simulink model "Q2_Model"  (R2021a)
settings: Solver=ode8  StartTime=0.0  StopTime=60  FixedStep=1e-4  RelTol=1e-3
InitFcn:
  | MagicFormula
  | LookUpTable
  | Q2_constants
values from neighbouring files (symbols this model uses):
  engine_torque = [-40 -44 -49 -53 -57 -61 -65 -70 -74 -78 -82 ... (first row only)    [LookUpTable.m]
  Je = 0.7    [Q2_constants.m]
  Jw = 0.7    [Q2_constants.m]
  MagicTire_Fx = Fx    [MagicFormula.m]
  MagicTire_Fy = Fy    [MagicFormula.m]
  MagicTire_Fz = 2000:2000:8000    [MagicFormula.m]
  Reff = 0.315    [Q2_constants.m]
  throt_angle = [0, 20, 30, 40, 50, 60, 70, 80, 90, 100]    [LookUpTable.m]
  whel_rot_angle = [83.70, 125.6, 167.5, 209.4, 251.3, 293.2, 335.1, 377.0, 418.9, 460.7, 502.6]    [LookUpTable.m]
undefined symbols (not defined in the file or in its folder): sigbuilder_block
libraries: pid_lib x1
settings Model: Creator=Fatih  LastModifiedBy=Fatih
settings DataIOCC: ReturnWorkspaceOutputs=off

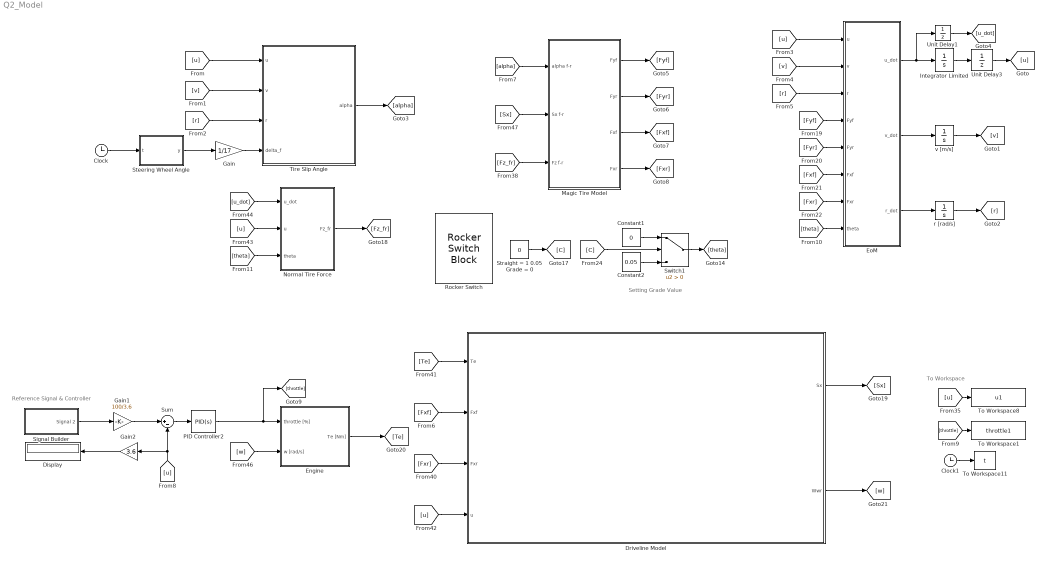
== system Q2_Model ==
  note: Reference Signal & Controller
  note: To Workspace
  note: Setting Grade Value
  Clock : Clock
  Clock1 : Clock
  Constant1 : Constant  Value=0
  Constant2 : Constant  Value=0.05
  Display : Display
  Driveline Model : Subsystem
  Engine : Subsystem
  EoM : MATLAB Function  TreatAsAtomicUnit=on
  Gain : Gain  Gain=1/17
  Gain1 : Gain  Gain=100/3.6
  Gain2 : Gain  Gain=3.6
  Integrator Limited : Integrator  InitialCondition=60/3.6  LimitOutput=on  UpperSaturationLimit=500  LowerSaturationLimit=1
  Magic Tire Model : Subsystem
  Normal Tire Force : MATLAB Function  TreatAsAtomicUnit=on
  PID Controller2 : pid_lib/PID Controller  Controller=PID  Form=Parallel  TimeDomain=Continuous-time  UseExternalTs=off  SampleTime=-1  IntegratorMethod=Forward Euler  FilterMethod=Forward Euler  ControllerParametersSource=internal  P=11  I=0.12  D=4  UseFilter=on  N=100  TunerSelectOption=Frequency Response Based  InitialConditionSource=internal  InitialConditionForIntegrator=0  InitialConditionForFilter=0  DifferentiatorICPrevScaledInput=0  ExternalReset=none  TrackingMode=off  Kt=1  LimitOutput=on  SatLimitsSource=internal  UpperSaturationLimit=90  LowerSaturationLimit=0  LinearizeAsGain=on  AntiWindupMode=none  Kb=1  POutMin=[]  POutMax=[]  IOutMin=[]  IOutMax=[]  DOutMin=[]  DOutMax=[]  NOutMin=[]  NOutMax=[]  SumOutMin=[]  SumOutMax=[]  SaturationOutMin=[]  SaturationOutMax=[]  PParamMin=[]  PParamMax=[]  IParamMin=[]  IParamMax=[]  DParamMin=[]  DParamMax=[]  NParamMin=[]  NParamMax=[]  KbParamMin=[]  KbParamMax=[]  KtParamMin=[]  KtParamMax=[]  KbOutMin=[]  KbOutMax=[]  KtOutMin=[]  KtOutMax=[]  IntegratorOutMin=[]  IntegratorOutMax=[]  FilterOutMin=[]  FilterOutMax=[]  SumI1OutMin=[]  SumI1OutMax=[]  SumI2OutMin=[]  SumI2OutMax=[]  SumI3OutMin=[]  SumI3OutMax=[]  SumI4OutMin=[]  SumI4OutMax=[]  SumDOutMin=[]  SumDOutMax=[]  DifferentiatorOutMin=[]  DifferentiatorOutMax=[]  FilterDiffOutCoefMin=[]  FilterDiffOutCoefMax=[]  ReciprocalOutMin=[]  ReciprocalOutMax=[]  SumDenOutMin=[]  SumDenOutMax=[]  SumNumOutMin=[]  SumNumOutMax=[]  DivideOutMin=[]  DivideOutMax=[]  UdiffTsProdOutMin=[]  UdiffTsProdOutMax=[]  NTsProdOutMin=[]  NTsProdOutMax=[]  UintegralTsProdOutMin=[]  UintegralTsProdOutMax=[]  UngainTsProdOutMin=[]  UngainTsProdOutMax=[]  IntegratorContinuousStateAttributes=''  IntegratorStateMustResolveToSignalObject=off  IntegratorRTWStateStorageClass=Auto  FilterContinuousStateAttributes=''  FilterStateMustResolveToSignalObject=off  FilterRTWStateStorageClass=Auto  ParallelPVariant=InternalParameters  IdealPVariant=Disabled  IVariant=InternalParameters  DVariant=InternalParameters  IntegratorVariant=Continuous  SatVariant=Enabled  AWVariant=Passthrough  PCopyVariant=Disabled  TRVariant=Disabled  FdbkBlocksVariant=Forward  IdealPFdbkVariant=Disabled  SatFdbkVariant=Disabled  DerivativeFilterVariant=ContFilter  NVariant=InternalParameters  NCopyVariant=Disabled  FilterICVariant=InternalICsFilter  IntegratorICVariant=InternalICs  ExternalResetVariant=Disabled  TRSumVariant=Passthrough  SumFdbkVariant=Disabled  SumVariant=Sum_PID  TsampFilterVariant=InternalTs  TsampNgainVariant=Passthrough  TsampIntegralVariant=Passthrough  ExternalSaturationOutDataTypeStr=Inherit: Same as second input
  Rocker Switch : RockerSwitchBlock
      settings: Values={{'Off', 'On'}, [0 1]}
  Signal Builder : Subsystem  Tag=STV Subsys  LoadFcn=sigbuilder_block('load');  StartFcn=sigbuilder_block('start');  StopFcn=sigbuilder_block('stop');  ClipboardFcn=sigbuilder_block('clipboard');  mask(Sigbuilder block){tuvar=[0:10]}
      mask help: Simulink:masks:SigbuilderBlock_MD
      mask init:
      | if ~strcmp(get_param(bdroot(gcbh),'SimulationStatus'),'stopped') tuvar = sigbuilder_block('maskInit'); end
      settings: CopyFcn=sigbuilder_block('copy');  DeleteFcn=sigbuilder_block('delete');  ModelCloseFcn=sigbuilder_block('modelClose');  PreSaveFcn=sigbuilder_block('preSave');  PauseFcn=sigbuilder_block('pause');  ContinueFcn=sigbuilder_block('continue');  NameChangeFcn=sigbuilder_block('namechange');  OpenFcn=sigbuilder_block('open',[437.6 199.2 550.4 400 ]);  CloseFcn=sigbuilder_block('close');
      mask Display: plot(0, 0, 100, 100,[2, 2, 32, 32, 2], [68, 8, 8, 68, 68],[32, 2], [38, 38], [32, 19, 2],[53, 60, 44], [32, 17, 17, 2],[16, 16, 31, 31]);txt = getActiveGroup(gcbh);text(2, 100, txt,'verticalAlignment', 'top');
  Steering Wheel Angle : MATLAB Function  TreatAsAtomicUnit=on
  Straight = 1 0.05 Grade = 0 : Constant  Value=0
  Sum : Sum  Inputs=|+-
  Switch1 : Switch  Criteria=u2 > Threshold
  Tire Slip Angle : MATLAB Function  TreatAsAtomicUnit=on
  To Workspace1 : ToWorkspace  VariableName=throttle1  SaveFormat=Timeseries  SampleTime=-1
      settings: Save2DSignal=2-D array (concatenate along first dimension)
  To Workspace11 : ToWorkspace  VariableName=t  SampleTime=-1
      settings: Save2DSignal=2-D array (concatenate along first dimension)
  To Workspace8 : ToWorkspace  VariableName=u1  SaveFormat=Timeseries  SampleTime=-1
      settings: Save2DSignal=2-D array (concatenate along first dimension)
  Unit Delay1 : UnitDelay  InitialCondition=1  SampleTime=-1  HasFrameUpgradeWarning=on
  Unit Delay3 : UnitDelay  InitialCondition=1  SampleTime=-1  HasFrameUpgradeWarning=on
  r [rad/s] : Integrator  InitialCondition=0.001
  v [m/s] : Integrator
  wires:
  Gain/1 -> Tire Slip Angle/4(delta_f)
  EoM/2(v_dot) -> v [m/s]/1
  EoM/3(r_dot) -> r [rad/s]/1
  v [m/s]/1 -> [v]
  r [rad/s]/1 -> [r]
  [u] -> Tire Slip Angle/1(u)
  [v] -> Tire Slip Angle/2(v)
  [r] -> Tire Slip Angle/3(r)
  [u] -> EoM/1(u)
  [r] -> EoM/3(r)
  Integrator Limited/1 -> Unit Delay3/1
  Clock/1 -> Steering Wheel Angle/1(t)
  Steering Wheel Angle/1(y) -> Gain/1
  Engine/1(Te [Nm]) -> [Te]
  Tire Slip Angle/1(alpha) -> [alpha]
  [alpha] -> Magic Tire Model/1(alpha f-r)
  [Sx] -> Magic Tire Model/2(Sx f-r)
  Magic Tire Model/3(Fxf) -> [Fxf]
  Magic Tire Model/2(Fyr) -> [Fyr]
  Magic Tire Model/1(Fyf) -> [Fyf]
  [Fyf] -> EoM/4(Fyf)
  [Fyr] -> EoM/5(Fyr)
  [Fxf] -> EoM/6(Fxf)
  [Fxr] -> EoM/7(Fxr)
  [u] -> To Workspace8/1
  Clock1/1 -> To Workspace11/1
  [Fz_fr] -> Magic Tire Model/3(Fz f-r)
  Magic Tire Model/4(Fxr) -> [Fxr]
  [w] -> Engine/2(w [rad/s])
  Unit Delay3/1 -> [u]
  [u] -> Sum/2, Gain2/1
  Signal Builder/1(Signal 2) -> Gain1/1
  Gain1/1 -> Sum/1
  Gain2/1 -> Display/1
  [Te] -> Driveline Model/1(Te)
  [Fxf] -> Driveline Model/2(Fxf)
  [Fxr] -> Driveline Model/3(Fxr)
  [u] -> Driveline Model/4(u)
  Driveline Model/1(Sx) -> [Sx]
  Driveline Model/2(Wwr) -> [w]
  [u] -> Normal Tire Force/2(u)
  [u_dot] -> Normal Tire Force/1(u_dot)
  Normal Tire Force/1(Fz_fr) -> [Fz_fr]
  PID Controller2/1 -> [throttle], Engine/1(throttle [%])
  Sum/1 -> PID Controller2/1
  EoM/1(u_dot) -> Unit Delay1/1, Integrator Limited/1
  Unit Delay1/1 -> [u_dot]
  [throttle] -> To Workspace1/1
  [v] -> EoM/2(v)
  Switch1/1 -> [theta]
  Constant2/1 -> Switch1/3
  [C] -> Switch1/2
  Straight = 1 0.05 Grade = 0/1 -> [C]
  Constant1/1 -> Switch1/1
  [theta] -> EoM/8(theta)
  [theta] -> Normal Tire Force/3(theta)

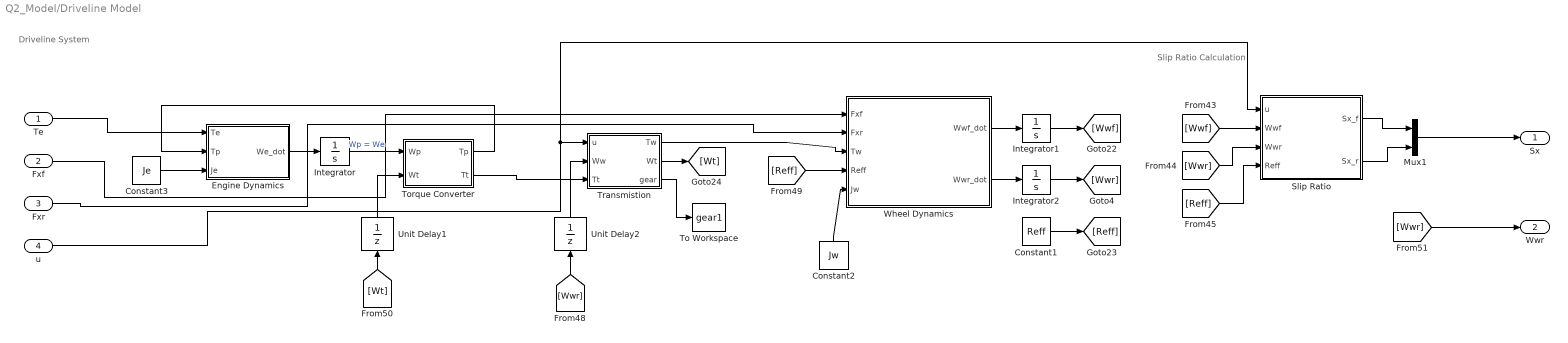
== system Q2_Model/Driveline Model ==
  note: Slip Ratio Calculation
  note: Driveline System
  Te : Inport
  Fxf : Inport  Port=2
  Fxr : Inport  Port=3
  u : Inport  Port=4
  Constant1 : Constant  Value=Reff
  Constant2 : Constant  Value=Jw
  Constant3 : Constant  Value=Je
  Engine Dynamics : MATLAB Function  TreatAsAtomicUnit=on
  Integrator : Integrator
  Integrator1 : Integrator  InitialCondition=100
  Integrator2 : Integrator  InitialCondition=100
  Mux1 : Mux  Inputs=2
  Slip Ratio : MATLAB Function  TreatAsAtomicUnit=on
  To Workspace : ToWorkspace  VariableName=gear1  SaveFormat=Timeseries  SampleTime=-1
  Torque Converter : MATLAB Function  TreatAsAtomicUnit=on
  Transmistion : MATLAB Function  TreatAsAtomicUnit=on
  Unit Delay1 : UnitDelay  InitialCondition=1  SampleTime=-1  HasFrameUpgradeWarning=on
  Unit Delay2 : UnitDelay  InitialCondition=1  SampleTime=-1  HasFrameUpgradeWarning=on
  Wheel Dynamics : MATLAB Function  TreatAsAtomicUnit=on
  Sx : Outport
  Wwr : Outport  Port=2
  wires:
  Engine Dynamics/1(We_dot) -> Integrator/1
  [Reff] -> Wheel Dynamics/4(Reff)
  [Wt] -> Unit Delay1/1
  u/1 -> Transmistion/1(u), Slip Ratio/1(u)
  [Wwr] -> Unit Delay2/1
  Integrator1/1 -> [Wwf]
  Unit Delay2/1 -> Transmistion/2(Ww)
  Transmistion/2(Wt) -> [Wt]
  Integrator2/1 -> [Wwr]
  Slip Ratio/1(Sx_f) -> Mux1/1
  Integrator/1 -> Torque Converter/1(Wp)  "Wp = We"
  [Wwf] -> Slip Ratio/2(Wwf)
  Slip Ratio/2(Sx_r) -> Mux1/2
  Constant1/1 -> [Reff]
  Unit Delay1/1 -> Torque Converter/2(Wt)
  Constant2/1 -> Wheel Dynamics/5(Jw)
  Fxr/1 -> Wheel Dynamics/2(Fxr)
  Wheel Dynamics/2(Wwr_dot) -> Integrator2/1
  [Wwr] -> Slip Ratio/3(Wwr)
  Torque Converter/1(Tp) -> Engine Dynamics/2(Tp)
  Transmistion/1(Tw) -> Wheel Dynamics/3(Tw)
  Constant3/1 -> Engine Dynamics/3(Je)
  [Reff] -> Slip Ratio/4(Reff)
  Wheel Dynamics/1(Wwf_dot) -> Integrator1/1
  Mux1/1 -> Sx/1
  [Wwr] -> Wwr/1
  Fxf/1 -> Wheel Dynamics/1(Fxf)
  Te/1 -> Engine Dynamics/1(Te)
  Transmistion/3(gear) -> To Workspace/1
  Torque Converter/2(Tt) -> Transmistion/3(Tt)

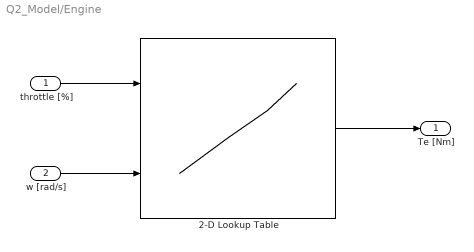
== system Q2_Model/Engine ==
  throttle [%] : Inport
  w [rad/s] : Inport  Port=2
  2-D Lookup Table : Lookup_n-D  BreakpointsForDimension1=throt_angle  BreakpointsForDimension2=whel_rot_angle  Table=engine_torque  InternalRulePriority=Speed  RndMeth=Simplest  InputSameDT=on
      settings: InputPortMap=u0,u1
  Te [Nm] : Outport
  wires:
  2-D Lookup Table/1 -> Te [Nm]/1
  throttle [%]/1 -> 2-D Lookup Table/1
  w [rad/s]/1 -> 2-D Lookup Table/2

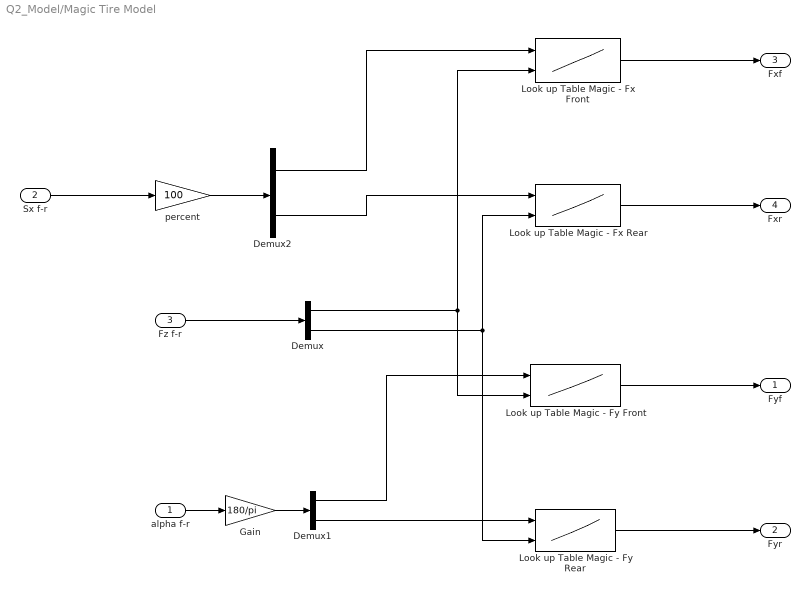
== system Q2_Model/Magic Tire Model ==
  alpha f-r : Inport
  Sx f-r : Inport  Port=2
  Fz f-r : Inport  Port=3
  Demux : Demux  Outputs=2
  Demux1 : Demux  Outputs=2
  Demux2 : Demux  Outputs=2
  Gain : Gain  Gain=180/pi
  Look up Table Magic - Fx Front : Lookup_n-D  BreakpointsForDimension1=MagicTire_slip_ratio'  BreakpointsForDimension2=MagicTire_Fz  Table=MagicTire_Fx  InternalRulePriority=Speed  RndMeth=Simplest  InputSameDT=on
      settings: InputPortMap=u0,u1
  Look up Table Magic - Fx Rear : Lookup_n-D  BreakpointsForDimension1=MagicTire_slip_ratio'  BreakpointsForDimension2=MagicTire_Fz  Table=MagicTire_Fx  InternalRulePriority=Speed  RndMeth=Simplest  InputSameDT=on
      settings: InputPortMap=u0,u1
  Look up Table Magic - Fy Front : Lookup_n-D  BreakpointsForDimension1=MagicTire_alpha'  BreakpointsForDimension2=MagicTire_Fz  Table=MagicTire_Fy  InternalRulePriority=Speed  RndMeth=Simplest  InputSameDT=on
      settings: InputPortMap=u0,u1
  Look up Table Magic - Fy Rear : Lookup_n-D  BreakpointsForDimension1=MagicTire_alpha'  BreakpointsForDimension2=MagicTire_Fz  Table=MagicTire_Fy  InternalRulePriority=Speed  RndMeth=Simplest  InputSameDT=on
      settings: InputPortMap=u0,u1
  percent : Gain  Gain=100
  Fyf : Outport
  Fyr : Outport  Port=2
  Fxf : Outport  Port=3
  Fxr : Outport  Port=4
  wires:
  Gain/1 -> Demux1/1
  Demux/1 -> Look up Table Magic - Fy Front/2, Look up Table Magic - Fx Front/2
  Sx f-r/1 -> percent/1
  alpha f-r/1 -> Gain/1
  Demux1/2 -> Look up Table Magic - Fy Rear/1
  Demux1/1 -> Look up Table Magic - Fy Front/1
  Demux/2 -> Look up Table Magic - Fy Rear/2, Look up Table Magic - Fx Rear/2
  Fz f-r/1 -> Demux/1
  Look up Table Magic - Fx Front/1 -> Fxf/1
  Look up Table Magic - Fx Rear/1 -> Fxr/1
  Look up Table Magic - Fy Front/1 -> Fyf/1
  Look up Table Magic - Fy Rear/1 -> Fyr/1
  percent/1 -> Demux2/1
  Demux2/2 -> Look up Table Magic - Fx Rear/1
  Demux2/1 -> Look up Table Magic - Fx Front/1

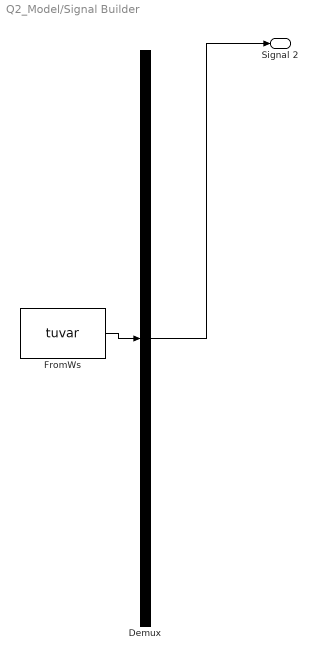
== system Q2_Model/Signal Builder ==
  Demux : Demux  Tag=STV Demux  Outputs=1
      settings: DisplayOption=none
  FromWs : FromWorkspace  Tag=STV FromWs  VariableName=tuvar
      SigBuilderData=|
      | common.afterFinalStr = 'Extrapolate'
      | common.sampleTime = 0
      | dataSet.timeRange = [0 80]
      | dataSet.name = 'Group 1'
      | sbobj.Groups.Name = 'Group 1'
      | sbobj.Groups.Signals.Name = 'Signal 2'
      | sbobj.Groups.Signals.XData = [0 10 10 30 30 80]
      | sbobj.Groups.Signals.YData = [0.6 0.6 1 1 0.4 0.4]
      | sbobj.Groups.TimeRange = [0 80]
  Signal 2 : Outport  Tag=STV Outport
  wires:
  FromWs/1 -> Demux/1
  Demux/1 -> Signal 2/1

== matlab function Q2_Model/Tire Slip Angle ==
  data: u input; alpha output; v input; r input; delta_f input
function alpha  = fcn(u,v,r,delta_f)

%Constants
lf = 1421e-03;  %longitudinal distance from c.g. to FREONT tires
lr = 1029e-03; %longitudinal distance from c.g. to REAR tires


alpha_f = delta_f -((v+lf*r)/u);    %Tire Slip angle front (eq:2.23 and eq:2.29 @ Rajesh Rajamani’s book)

alpha_r =  -((v-lr*r)/u);           %Tire Slip angle rear (eq:2.24 and eq:2.30 @ Rajesh Rajamani’s book)

alpha=[alpha_f,alpha_r];

== matlab function Q2_Model/Normal Tire Force ==
  data: u_dot input; Fz_fr output; u input; theta input
function Fz_fr = fcn(u_dot,u,theta)

% Constants
m = 1480; % kg
g = 9.81; % m/s^2
lf = 1421*10^-3; % m
lr = 1029*10^-3; % m
h_g = 420*10^-3; % m
h_aero = 1.2*h_g; % m (assumption)

rho = 1.225; % kg/m^3
Cd = 0.335;
Area_front = 1.824; % m^2
F_aero = 0.5*rho*Cd*Area_front*u^2;

Fzf = ((-F_aero*h_aero)-(m*u_dot*h_g)-(m*g*h_g*sin(theta))+(m*g*lr*cos(theta)))/(lf+lr);
Fzr = ((F_aero*h_aero)+(m*u_dot*h_g)-(m*g*h_g*sin(theta))+(m*g*lf*cos(theta)))/(lf+lr);

Fz_fr = [Fzf Fzr];

== matlab function Q2_Model/EoM ==
  data: u input; v input; u_dot output; r input; Fyf input; Fyr input; v_dot output; r_dot output; Fxf input; Fxr input; theta input
function [u_dot,v_dot,r_dot] = fcn(u,v,r,Fyf,Fyr,Fxf,Fxr,theta)

%% constants
Jz = 1950;          %[kgm^2]
lf = 1421*10^-3;     %[m] 
lr = 1029*10^-3;    %[m]

%% Aerodynamic Force
rho = 1.225;                        %[kg/m^2]
Cd = 0.335;                          %
Area_front = 1.824;       %[m^2]

% Rolling resistance
m = 1480;                            %[kg]
g = 9.81;                           %[m/s^2]
f0 = 0.013;                         %
Fr = f0*(m*g)/2;                    %[N]

%% Equation of Motions

v_dot = (Fyf + Fyr)/m - r*u;    %Vd&C Eq(2.21)

r_dot = (lf*Fyf - lr*Fyr)/Jz;   %Vd&C Eq(2.22)

Faero = 0.5*rho*Cd*Area_front*u^2;

u_dot = (Fxf + Fxr - Fr - Faero - m*g*sin(theta))/m;

== matlab function Q2_Model/Steering Wheel Angle ==
  data: t input; y output
function y = fcn(t)

y = 0*t;

== matlab function Q2_Model/Driveline Model/Engine Dynamics ==
  data: Te input; We_dot output; Tp input; Je input
function We_dot  = fcn(Te,Tp,Je)

We_dot = (Te-Tp)/Je;

== matlab function Q2_Model/Driveline Model/Slip Ratio ==
  data: u input; Sx_f output; Wwf input; Wwr input; Reff input; Sx_r output
function [Sx_f,Sx_r] = fcn(u,Wwf,Wwr,Reff)

Sx_f = ((Reff*Wwf)-u)/(Reff*Wwf); %Slip ratio (eq:4.12)
Sx_r = ((Reff*Wwr)-u)/(Reff*Wwr);

== matlab function Q2_Model/Driveline Model/Torque Converter ==
  data: Wp input; Tp output; Wt input; Tt output
function [Tp,Tt] = fcn(Wp,Wt)


%for converting mode

if Wt/Wp < 0.9
    Tp = (3.43e-03*Wp^2)+(2.22e-03*Wp*Wt)-(4.6e-03*Wt^2);       % Eq 4.28 @ Rajamani
    Tt = (5.77e-03*Wp^2)+(0.31e-03*Wp*Wt)-(5.43e-03*Wt^2);      % Eq 4.29 @ Rajamani

%for fuild coupling mode (Wt/Wp >= 0.9)

else
    
    Tp = (-6.76e-03*Wp^2)+(32e-03*Wp*Wt)-(25.24e-03*Wt^2);      % Eq 4.30 @ Rajamani
    Tt = Tp;
end

end

== matlab function Q2_Model/Driveline Model/Transmistion ==
  data: u input; Tw output; Ww input; Tt input; Wt output; gear output
function [Tw,Wt,gear] = fcn(u,Ww,Tt)

gear=0;
N = [(1/3.214) (1/2.105) (1/1.458) (1/1.094) (1/0.861)];
Nf = 1/ 4.051;

if u >= 0 && u <= (25/3.6) 
    gear = 1;
    Tfd = Tt/N(1);
    Tw = Tfd/Nf;

    Wfd = Ww/N(2);
    Wt = Wfd/Nf;

elseif u > (25/3.6) && u <= (45/3.6)
    gear = 2;
    Tfd = Tt/N(2);
    Tw = Tfd/Nf;

    Wfd = Ww/N(2);
    Wt = Wfd/Nf;

elseif u > (45/3.6) && u <= (75/3.6)
    gear = 3;
    Tfd = Tt/N(3);
    Tw = Tfd/Nf;

    Wfd = Ww/N(3);
    Wt = Wfd/Nf;

elseif u > (75/3.6) && u <= (95/3.6)
    gear = 4;
    Tfd = Tt/N(4);
    Tw = Tfd/Nf;

    Wfd = Ww/N(4);
    Wt = Wfd/Nf;

elseif u > (95/3.6) && u <= (240/3.6)
    gear = 5;
    Tfd = Tt/N(5);
    Tw = Tfd/Nf;

    Wfd = Ww/N(5);
    Wt = Wfd/Nf;

else
    Tw =0;
    Wt =0; 
end

== matlab function Q2_Model/Driveline Model/Wheel Dynamics ==
  data: Fxf input; Wwf_dot output; Fxr input; Tw input; Reff input; Jw input; Wwr_dot output
function [Wwf_dot,Wwr_dot] = fcn(Fxf,Fxr,Tw,Reff,Jw)

Wwf_dot = (-Reff*Fxf)/Jw;
Wwr_dot = (Tw-Reff*Fxr)/Jw;
